simulink model "PHAT"  (Simulink 6.5)
settings: Solver=FixedStepDiscrete  StartTime=0.0  StopTime=0.0  FixedStep=1  RelTol=1e-3
undefined symbols (not defined in the file): magnitude
libraries: dspxfrm3 x28, dspsigops x7
settings Model: Creator=eettinger  LastModifiedBy=cameraman  ExtModeAutoUpdateStatusClock=off
settings OptimizationCC: OptimizeModelRefInitCode=on  LifeSpan=1
settings RTWCC: SystemTargetFile=ert.tlc  TemplateMakefile=ert_default_tmf  Description=Real-Time Workshop Embedded Coder (no auto configuration)  GenerateReport=on  ProcessScript=ert_make_rtw_hook  IncludeHyperlinkInReport=on  LaunchReport=on
settings CodeAppCC: IgnoreCustomStorageClasses=off
settings ERTTargetCC: TargetFcnLib=ansi_tfl_tmw.mat  GenFloatMathFcnCalls=ANSI_C  GenerateSampleERTMain=on  InlinedParameterPlacement=NonHierarchical  ERTCustomFileTemplate=example_file_process.tlc

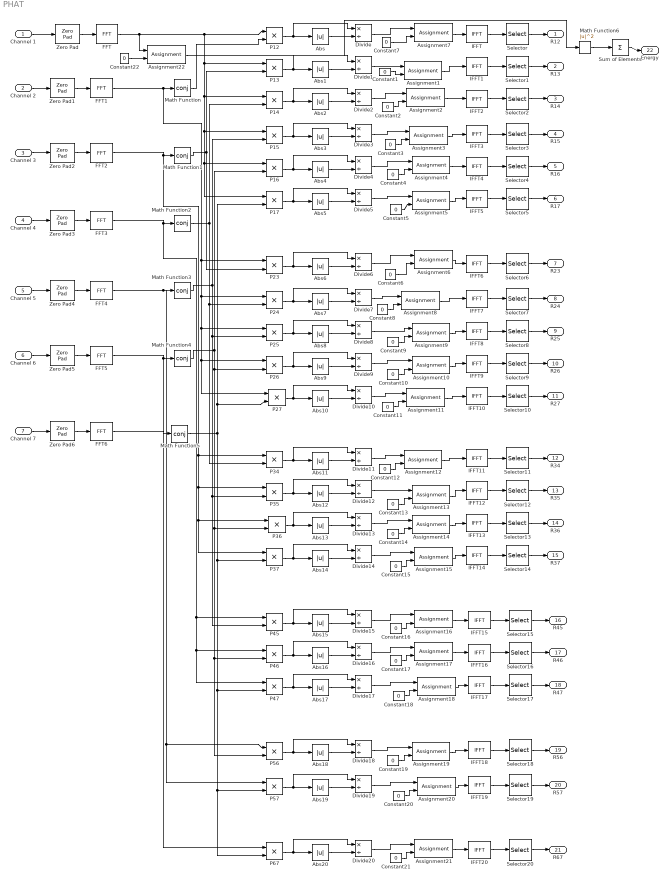
== system PHAT ==
  Channel 1 : Inport  PortDimensions=[1600 1]  DataType=single
  Channel 2 : Inport  Port=2  PortDimensions=[1600 1]  DataType=single
  Channel 3 : Inport  Port=3  PortDimensions=[1600 1]  DataType=single
  Channel 4 : Inport  Port=4  PortDimensions=[1600 1]  DataType=single
  Channel 5 : Inport  Port=5  PortDimensions=[1600 1]  DataType=single
  Channel 6 : Inport  Port=6  PortDimensions=[1600 1]  DataType=single
  Channel 7 : Inport  Port=7  PortDimensions=[1600 1]  DataType=single
  Abs{,1..20} (21 alike) : Abs
  Assignment{1..22} (22 alike) : Assignment  InputType=Vector  IndexIsStartValue=off  ElementSrc=Internal  Elements=[2:64,1986:2048]  RowSrc=Internal  Rows=1  ColumnSrc=Internal  Columns=1  OutputInitialize=Initialize using input (U1)  OutputDimensions=[1 1]
  Constant{1..22} (22 alike) : Constant  Value=0  OutDataTypeMode=single
  Divide{,1..20} (21 alike) : Product  Inputs=*/  OutScaling=2^-10
  FFT : dspxfrm3/FFT  DialogController=dspDDGCreate  DialogControllerArgs=DataTag0  CompMethod=Table lookup  TableOpt=Speed  BitRevOrder=off  SkipNorm=on  roundingMode=Floor  overflowMode=off
  FFT1 : dspxfrm3/FFT  DialogController=dspDDGCreate  DialogControllerArgs=DataTag1  CompMethod=Table lookup  TableOpt=Speed  BitRevOrder=off  SkipNorm=on  roundingMode=Floor  overflowMode=off
  FFT2 : dspxfrm3/FFT  DialogController=dspDDGCreate  DialogControllerArgs=DataTag2  CompMethod=Table lookup  TableOpt=Speed  BitRevOrder=off  SkipNorm=on  roundingMode=Floor  overflowMode=off
  FFT3 : dspxfrm3/FFT  DialogController=dspDDGCreate  DialogControllerArgs=DataTag3  CompMethod=Table lookup  TableOpt=Speed  BitRevOrder=off  SkipNorm=on  roundingMode=Floor  overflowMode=off
  FFT4 : dspxfrm3/FFT  DialogController=dspDDGCreate  DialogControllerArgs=DataTag4  CompMethod=Table lookup  TableOpt=Speed  BitRevOrder=off  SkipNorm=on  roundingMode=Floor  overflowMode=off
  FFT5 : dspxfrm3/FFT  DialogController=dspDDGCreate  DialogControllerArgs=DataTag5  CompMethod=Table lookup  TableOpt=Speed  BitRevOrder=off  SkipNorm=on  roundingMode=Floor  overflowMode=off
  FFT6 : dspxfrm3/FFT  DialogController=dspDDGCreate  DialogControllerArgs=DataTag6  CompMethod=Table lookup  TableOpt=Speed  BitRevOrder=off  SkipNorm=on  roundingMode=Floor  overflowMode=off
  IFFT : dspxfrm3/IFFT  DialogController=dspDDGCreate  DialogControllerArgs=DataTag7  CompMethod=Table lookup  TableOpt=Speed  BitRevOrder=off  cs_in=on  SkipNorm=off  mode=Complex  roundingMode=Floor  overflowMode=off
  IFFT1 : dspxfrm3/IFFT  DialogController=dspDDGCreate  DialogControllerArgs=DataTag8  CompMethod=Table lookup  TableOpt=Speed  BitRevOrder=off  cs_in=on  SkipNorm=off  mode=Complex  roundingMode=Floor  overflowMode=off
  IFFT10 : dspxfrm3/IFFT  DialogController=dspDDGCreate  DialogControllerArgs=DataTag9  CompMethod=Table lookup  TableOpt=Speed  BitRevOrder=off  cs_in=on  SkipNorm=off  mode=Complex  roundingMode=Floor  overflowMode=off
  IFFT11 : dspxfrm3/IFFT  DialogController=dspDDGCreate  DialogControllerArgs=DataTag10  CompMethod=Table lookup  TableOpt=Speed  BitRevOrder=off  cs_in=on  SkipNorm=off  mode=Complex  roundingMode=Floor  overflowMode=off
  IFFT12 : dspxfrm3/IFFT  DialogController=dspDDGCreate  DialogControllerArgs=DataTag11  CompMethod=Table lookup  TableOpt=Speed  BitRevOrder=off  cs_in=on  SkipNorm=off  mode=Complex  roundingMode=Floor  overflowMode=off
  IFFT13 : dspxfrm3/IFFT  DialogController=dspDDGCreate  DialogControllerArgs=DataTag12  CompMethod=Table lookup  TableOpt=Speed  BitRevOrder=off  cs_in=on  SkipNorm=off  mode=Complex  roundingMode=Floor  overflowMode=off
  IFFT14 : dspxfrm3/IFFT  DialogController=dspDDGCreate  DialogControllerArgs=DataTag13  CompMethod=Table lookup  TableOpt=Speed  BitRevOrder=off  cs_in=on  SkipNorm=off  mode=Complex  roundingMode=Floor  overflowMode=off
  IFFT15 : dspxfrm3/IFFT  DialogController=dspDDGCreate  DialogControllerArgs=DataTag14  CompMethod=Table lookup  TableOpt=Speed  BitRevOrder=off  cs_in=on  SkipNorm=off  mode=Complex  roundingMode=Floor  overflowMode=off
  IFFT16 : dspxfrm3/IFFT  DialogController=dspDDGCreate  DialogControllerArgs=DataTag15  CompMethod=Table lookup  TableOpt=Speed  BitRevOrder=off  cs_in=on  SkipNorm=off  mode=Complex  roundingMode=Floor  overflowMode=off
  IFFT17 : dspxfrm3/IFFT  DialogController=dspDDGCreate  DialogControllerArgs=DataTag16  CompMethod=Table lookup  TableOpt=Speed  BitRevOrder=off  cs_in=on  SkipNorm=off  mode=Complex  roundingMode=Floor  overflowMode=off
  IFFT18 : dspxfrm3/IFFT  DialogController=dspDDGCreate  DialogControllerArgs=DataTag17  CompMethod=Table lookup  TableOpt=Speed  BitRevOrder=off  cs_in=on  SkipNorm=off  mode=Complex  roundingMode=Floor  overflowMode=off
  IFFT19 : dspxfrm3/IFFT  DialogController=dspDDGCreate  DialogControllerArgs=DataTag18  CompMethod=Table lookup  TableOpt=Speed  BitRevOrder=off  cs_in=on  SkipNorm=off  mode=Complex  roundingMode=Floor  overflowMode=off
  IFFT2 : dspxfrm3/IFFT  DialogController=dspDDGCreate  DialogControllerArgs=DataTag19  CompMethod=Table lookup  TableOpt=Speed  BitRevOrder=off  cs_in=on  SkipNorm=off  mode=Complex  roundingMode=Floor  overflowMode=off
  IFFT20 : dspxfrm3/IFFT  DialogController=dspDDGCreate  DialogControllerArgs=DataTag20  CompMethod=Table lookup  TableOpt=Speed  BitRevOrder=off  cs_in=on  SkipNorm=off  mode=Complex  roundingMode=Floor  overflowMode=off
  IFFT3 : dspxfrm3/IFFT  DialogController=dspDDGCreate  DialogControllerArgs=DataTag21  CompMethod=Table lookup  TableOpt=Speed  BitRevOrder=off  cs_in=on  SkipNorm=off  mode=Complex  roundingMode=Floor  overflowMode=off
  IFFT4 : dspxfrm3/IFFT  DialogController=dspDDGCreate  DialogControllerArgs=DataTag22  CompMethod=Table lookup  TableOpt=Speed  BitRevOrder=off  cs_in=on  SkipNorm=off  mode=Complex  roundingMode=Floor  overflowMode=off
  IFFT5 : dspxfrm3/IFFT  DialogController=dspDDGCreate  DialogControllerArgs=DataTag23  CompMethod=Table lookup  TableOpt=Speed  BitRevOrder=off  cs_in=on  SkipNorm=off  mode=Complex  roundingMode=Floor  overflowMode=off
  IFFT6 : dspxfrm3/IFFT  DialogController=dspDDGCreate  DialogControllerArgs=DataTag24  CompMethod=Table lookup  TableOpt=Speed  BitRevOrder=off  cs_in=on  SkipNorm=off  mode=Complex  roundingMode=Floor  overflowMode=off
  IFFT7 : dspxfrm3/IFFT  DialogController=dspDDGCreate  DialogControllerArgs=DataTag25  CompMethod=Table lookup  TableOpt=Speed  BitRevOrder=off  cs_in=on  SkipNorm=off  mode=Complex  roundingMode=Floor  overflowMode=off
  IFFT8 : dspxfrm3/IFFT  DialogController=dspDDGCreate  DialogControllerArgs=DataTag26  CompMethod=Table lookup  TableOpt=Speed  BitRevOrder=off  cs_in=on  SkipNorm=off  mode=Complex  roundingMode=Floor  overflowMode=off
  IFFT9 : dspxfrm3/IFFT  DialogController=dspDDGCreate  DialogControllerArgs=DataTag27  CompMethod=Table lookup  TableOpt=Speed  BitRevOrder=off  cs_in=on  SkipNorm=off  mode=Complex  roundingMode=Floor  overflowMode=off
  Math Function{,1..5} (6 alike) : Math  Operator=conj  SaturateOnIntegerOverflow=on
  Math Function6 : Math  Operator=magnitude^2  SaturateOnIntegerOverflow=on
  P{12..17,23..27,34..37,45..47,56..57,67} (21 alike) : Product  RndMeth=Zero
  Selector{,1..20} (21 alike) : Selector  InputType=Vector  ElementSrc=Internal  Elements=[1548:2048 1:500]  RowSrc=Internal  Rows=1  ColumnSrc=Internal  Columns=1  IndexIsStartValue=off
  Sum of Elements : Sum  Inputs=+  OutScaling=2^-10
  Zero Pad : dspsigops/Zero Pad  DialogController=dspfixptddg.ZeroPad  DialogControllerArgs=DataTag28  padSigAt=End  zpadAlong=Columns  padNumOutRowsSpecMethod=Next power of two  numOutRows=1  padNumOutColsSpecMethod=Next power of two  numOutCols=1  truncOrWrapMode=Truncate  trunc_flag=None  wrap_flag=None  isVarDimsMode=off  roundingMode=Floor  overflowMode=off
  Zero Pad1 : dspsigops/Zero Pad  DialogController=dspfixptddg.ZeroPad  DialogControllerArgs=DataTag29  padSigAt=End  zpadAlong=Columns  padNumOutRowsSpecMethod=Next power of two  numOutRows=1  padNumOutColsSpecMethod=Next power of two  numOutCols=1  truncOrWrapMode=Truncate  trunc_flag=None  wrap_flag=None  isVarDimsMode=off  roundingMode=Floor  overflowMode=off
  Zero Pad2 : dspsigops/Zero Pad  DialogController=dspfixptddg.ZeroPad  DialogControllerArgs=DataTag30  padSigAt=End  zpadAlong=Columns  padNumOutRowsSpecMethod=Next power of two  numOutRows=1  padNumOutColsSpecMethod=Next power of two  numOutCols=1  truncOrWrapMode=Truncate  trunc_flag=None  wrap_flag=None  isVarDimsMode=off  roundingMode=Floor  overflowMode=off
  Zero Pad3 : dspsigops/Zero Pad  DialogController=dspfixptddg.ZeroPad  DialogControllerArgs=DataTag31  padSigAt=End  zpadAlong=Columns  padNumOutRowsSpecMethod=Next power of two  numOutRows=1  padNumOutColsSpecMethod=Next power of two  numOutCols=1  truncOrWrapMode=Truncate  trunc_flag=None  wrap_flag=None  isVarDimsMode=off  roundingMode=Floor  overflowMode=off
  Zero Pad4 : dspsigops/Zero Pad  DialogController=dspfixptddg.ZeroPad  DialogControllerArgs=DataTag32  padSigAt=End  zpadAlong=Columns  padNumOutRowsSpecMethod=Next power of two  numOutRows=1  padNumOutColsSpecMethod=Next power of two  numOutCols=1  truncOrWrapMode=Truncate  trunc_flag=None  wrap_flag=None  isVarDimsMode=off  roundingMode=Floor  overflowMode=off
  Zero Pad5 : dspsigops/Zero Pad  DialogController=dspfixptddg.ZeroPad  DialogControllerArgs=DataTag33  padSigAt=End  zpadAlong=Columns  padNumOutRowsSpecMethod=Next power of two  numOutRows=1  padNumOutColsSpecMethod=Next power of two  numOutCols=1  truncOrWrapMode=Truncate  trunc_flag=None  wrap_flag=None  isVarDimsMode=off  roundingMode=Floor  overflowMode=off
  Zero Pad6 : dspsigops/Zero Pad  DialogController=dspfixptddg.ZeroPad  DialogControllerArgs=DataTag34  padSigAt=End  zpadAlong=Columns  padNumOutRowsSpecMethod=Next power of two  numOutRows=1  padNumOutColsSpecMethod=Next power of two  numOutCols=1  truncOrWrapMode=Truncate  trunc_flag=None  wrap_flag=None  isVarDimsMode=off  roundingMode=Floor  overflowMode=off
  R12 : Outport  DataType=single
  R13 : Outport  Port=2  DataType=single
  R14 : Outport  Port=3  DataType=single
  R15 : Outport  Port=4  DataType=single
  R16 : Outport  Port=5  DataType=single
  R17 : Outport  Port=6  DataType=single
  R23 : Outport  Port=7  DataType=single
  R24 : Outport  Port=8  DataType=single
  R25 : Outport  Port=9  DataType=single
  R26 : Outport  Port=10  DataType=single
  R27 : Outport  Port=11  DataType=single
  R34 : Outport  Port=12  DataType=single
  R35 : Outport  Port=13  DataType=single
  R36 : Outport  Port=14  DataType=single
  R37 : Outport  Port=15  DataType=single
  R45 : Outport  Port=16  DataType=single
  R46 : Outport  Port=17  DataType=single
  R47 : Outport  Port=18  DataType=single
  R56 : Outport  Port=19  DataType=single
  R57 : Outport  Port=20  DataType=single
  R67 : Outport  Port=21  DataType=single
  Energy : Outport  Port=22  DataType=single
  wires:
  Zero Pad/1 -> FFT/1
  Zero Pad1/1 -> FFT1/1
  Zero Pad2/1 -> FFT2/1
  Zero Pad3/1 -> FFT3/1
  Zero Pad4/1 -> FFT4/1
  Zero Pad5/1 -> FFT5/1
  Zero Pad6/1 -> FFT6/1
  IFFT/1 -> Selector/1
  Selector/1 -> R12/1
  IFFT1/1 -> Selector1/1
  Selector1/1 -> R13/1
  IFFT2/1 -> Selector2/1
  Selector2/1 -> R14/1
  IFFT3/1 -> Selector3/1
  Selector3/1 -> R15/1
  IFFT4/1 -> Selector4/1
  Selector4/1 -> R16/1
  IFFT5/1 -> Selector5/1
  Selector5/1 -> R17/1
  IFFT6/1 -> Selector6/1
  Selector6/1 -> R23/1
  IFFT7/1 -> Selector7/1
  Selector7/1 -> R24/1
  IFFT8/1 -> Selector8/1
  Selector8/1 -> R25/1
  IFFT9/1 -> Selector9/1
  Selector9/1 -> R26/1
  IFFT10/1 -> Selector10/1
  Selector10/1 -> R27/1
  IFFT11/1 -> Selector11/1
  Selector11/1 -> R34/1
  IFFT12/1 -> Selector12/1
  Selector12/1 -> R35/1
  IFFT13/1 -> Selector13/1
  Selector13/1 -> R36/1
  IFFT14/1 -> Selector14/1
  Selector14/1 -> R37/1
  IFFT15/1 -> Selector15/1
  Selector15/1 -> R45/1
  IFFT16/1 -> Selector16/1
  Selector16/1 -> R46/1
  IFFT17/1 -> Selector17/1
  Selector17/1 -> R47/1
  IFFT18/1 -> Selector18/1
  Selector18/1 -> R56/1
  IFFT19/1 -> Selector19/1
  Selector19/1 -> R57/1
  IFFT20/1 -> Selector20/1
  Selector20/1 -> R67/1
  P12/1 -> Abs/1, Divide/1
  Abs/1 -> Divide/2
  P13/1 -> Abs1/1, Divide1/1
  Abs1/1 -> Divide1/2
  P14/1 -> Abs2/1, Divide2/1
  Abs2/1 -> Divide2/2
  P15/1 -> Abs3/1, Divide3/1
  Abs3/1 -> Divide3/2
  P16/1 -> Abs4/1, Divide4/1
  Abs4/1 -> Divide4/2
  P17/1 -> Abs5/1, Divide5/1
  Abs5/1 -> Divide5/2
  P23/1 -> Abs6/1, Divide6/1
  Abs6/1 -> Divide6/2
  P24/1 -> Abs7/1, Divide7/1
  Abs7/1 -> Divide7/2
  P25/1 -> Abs8/1, Divide8/1
  Abs8/1 -> Divide8/2
  P26/1 -> Abs9/1, Divide9/1
  Abs9/1 -> Divide9/2
  P27/1 -> Abs10/1, Divide10/1
  Abs10/1 -> Divide10/2
  P34/1 -> Abs11/1, Divide11/1
  Abs11/1 -> Divide11/2
  P35/1 -> Abs12/1, Divide12/1
  Abs12/1 -> Divide12/2
  P36/1 -> Abs13/1, Divide13/1
  Abs13/1 -> Divide13/2
  P37/1 -> Abs14/1, Divide14/1
  Abs14/1 -> Divide14/2
  P45/1 -> Abs15/1, Divide15/1
  Abs15/1 -> Divide15/2
  P46/1 -> Abs16/1, Divide16/1
  Abs16/1 -> Divide16/2
  P47/1 -> Abs17/1, Divide17/1
  Abs17/1 -> Divide17/2
  P56/1 -> Abs18/1, Divide18/1
  Abs18/1 -> Divide18/2
  P57/1 -> Abs19/1, Divide19/1
  Abs19/1 -> Divide19/2
  P67/1 -> Abs20/1, Divide20/1
  Abs20/1 -> Divide20/2
  Channel 1/1 -> Zero Pad/1
  Channel 7/1 -> Zero Pad6/1
  Channel 6/1 -> Zero Pad5/1
  Channel 5/1 -> Zero Pad4/1
  Channel 4/1 -> Zero Pad3/1
  Channel 3/1 -> Zero Pad2/1
  Channel 2/1 -> Zero Pad1/1
  FFT/1 -> P12/1, P13/1, P14/1, P15/1, P16/1, P17/1, Assignment22/1
  Math Function/1 -> P12/2
  FFT1/1 -> Math Function/1, P23/1, P24/1, P25/1, P26/1, P27/1
  FFT2/1 -> Math Function1/1, P34/1, P35/1, P36/1, P37/1
  FFT3/1 -> Math Function2/1, P45/1, P46/1, P47/1
  FFT4/1 -> Math Function3/1, P56/1, P57/1
  FFT5/1 -> Math Function4/1, P67/1
  FFT6/1 -> Math Function5/1
  Math Function1/1 -> P13/2, P23/2
  Math Function2/1 -> P14/2, P24/2, P34/2
  Math Function3/1 -> P15/2, P25/2, P35/2, P45/2
  Math Function4/1 -> P16/2, P26/2, P36/2, P46/2, P56/2
  Math Function5/1 -> P37/2, P47/2, P57/2, P67/2, P17/2, P27/2
  Constant7/1 -> Assignment7/2
  Divide/1 -> Assignment7/1
  Assignment7/1 -> IFFT/1
  Constant1/1 -> Assignment1/2
  Divide1/1 -> Assignment1/1
  Assignment1/1 -> IFFT1/1
  Constant2/1 -> Assignment2/2
  Divide2/1 -> Assignment2/1
  Assignment2/1 -> IFFT2/1
  Constant3/1 -> Assignment3/2
  Divide3/1 -> Assignment3/1
  Assignment3/1 -> IFFT3/1
  Constant4/1 -> Assignment4/2
  Divide4/1 -> Assignment4/1
  Assignment4/1 -> IFFT4/1
  Constant5/1 -> Assignment5/2
  Assignment5/1 -> IFFT5/1
  Divide5/1 -> Assignment5/1
  Constant6/1 -> Assignment6/2
  Assignment6/1 -> IFFT6/1
  Divide6/1 -> Assignment6/1
  Constant8/1 -> Assignment8/2
  Divide7/1 -> Assignment8/1
  Assignment8/1 -> IFFT7/1
  Constant9/1 -> Assignment9/2
  Divide8/1 -> Assignment9/1
  Assignment9/1 -> IFFT8/1
  Constant10/1 -> Assignment10/2
  Assignment10/1 -> IFFT9/1
  Divide9/1 -> Assignment10/1
  Constant11/1 -> Assignment11/2
  Divide10/1 -> Assignment11/1
  Assignment11/1 -> IFFT10/1
  Constant12/1 -> Assignment12/2
  Divide11/1 -> Assignment12/1
  Assignment12/1 -> IFFT11/1
  Constant13/1 -> Assignment13/2
  Divide12/1 -> Assignment13/1
  Assignment13/1 -> IFFT12/1
  Constant14/1 -> Assignment14/2
  Divide13/1 -> Assignment14/1
  Assignment14/1 -> IFFT13/1
  Constant15/1 -> Assignment15/2
  Divide14/1 -> Assignment15/1
  Assignment15/1 -> IFFT14/1
  Constant16/1 -> Assignment16/2
  Divide15/1 -> Assignment16/1
  Assignment16/1 -> IFFT15/1
  Constant17/1 -> Assignment17/2
  Divide16/1 -> Assignment17/1
  Assignment17/1 -> IFFT16/1
  Constant18/1 -> Assignment18/2
  Divide17/1 -> Assignment18/1
  Assignment18/1 -> IFFT17/1
  Constant19/1 -> Assignment19/2
  Divide18/1 -> Assignment19/1
  Assignment19/1 -> IFFT18/1
  Constant20/1 -> Assignment20/2
  Divide19/1 -> Assignment20/1
  Assignment20/1 -> IFFT19/1
  Constant21/1 -> Assignment21/2
  Divide20/1 -> Assignment21/1
  Assignment21/1 -> IFFT20/1
  Constant22/1 -> Assignment22/2
  Assignment22/1 -> Math Function6/1
  Sum of Elements/1 -> Energy/1
  Math Function6/1 -> Sum of Elements/1
